simulink model "testing_stuff_ej2"  (R2023b)
settings: Solver=VariableStepAuto  StartTime=0.0  StopTime=0.1  FixedStep=step  RelTol=1e-3
values from neighbouring files (symbols this model uses):
  ej3_offset = 1e-5    (= 1e-05)    [EJ3.m]
  fd = 10    [EJ3.m]
  Kenv = 1000000    [EJ3.m]
  Kp = wn^2    (= 21268.5764063)    [EJ3.m]
  Kpf = 160000*1000    (= 160000000)    [EJ3.m]
  Kv = eta*(2*sqrt(Kp))    [EJ3.m]
  Kvf = 800*sqrt(1000)    [EJ3.m]
  mask = [1 1 0 0 0 0]    [EJ3.m]
  q0 = [pi/2,-pi/2]    [EJ3.m]
  robot = SerialLink(L, 'tool', Tool)    [EJ3.m]
  WO_R2x2 = WO_T(1:2,1:2)    [EJ3.m]
  WO_T = trotz(-pi/4)*transl(-1,-1,0)    [EJ3.m]
undefined symbols (not defined in the file or in its folder): coriolis, fkine, friction, gravload, inertia, jacob0, subsref, transl
libraries: roblocks x2, matrix_library x2
settings Model: Creator=alero  LastModifiedBy=alero

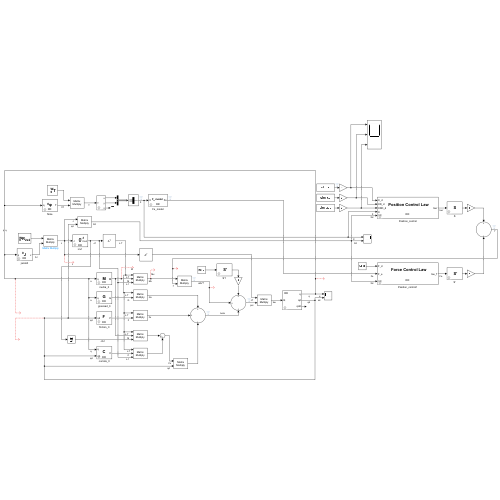
[thumbnail: Simulink's stored preview of the top-level diagram]
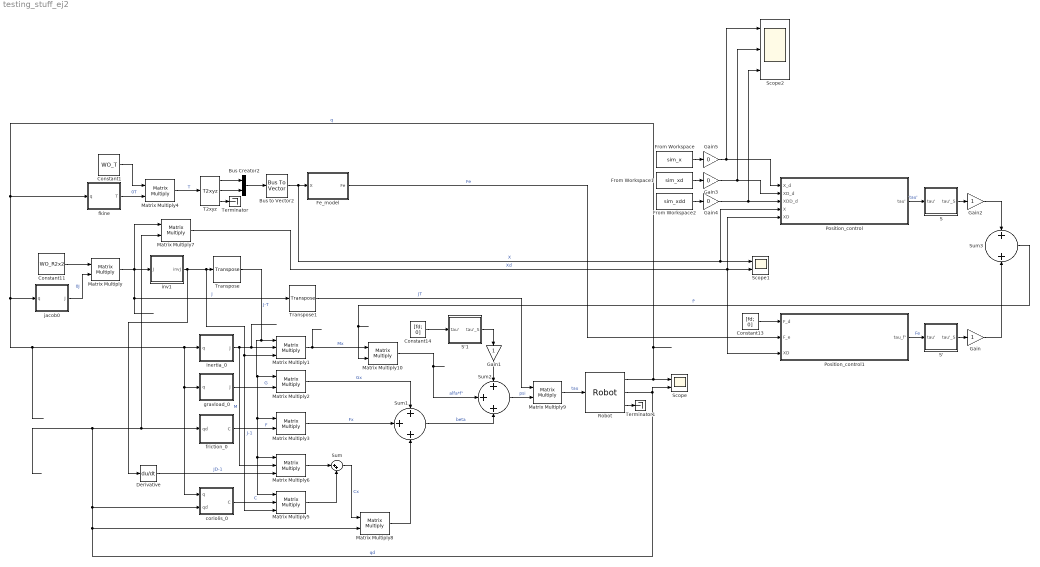
== system testing_stuff_ej2 ==
  Bus Creator2 : BusCreator  Inputs=2
  Bus to Vector2 : BusToVector
  Constant1 : Constant  Value=WO_T  VectorParams1D=off
      mask Display:
      | text(0.35, 0.8, '\bf\fontsize{16}^W_0T', 'texmode', 'on', 'verticalAlignment', 'top', 'horizontalAlignment', 'left')
      | %text(0.45, 0.65, '\fontsize{10}0', 'texmode', 'on','verticalAlignment', 'bottom', 'horizontalAlignment', 'right')
  Constant11 : Constant  Value=WO_R2x2  VectorParams1D=off
      mask Display:
      | text(0.1, 0.8, '\bf\fontsize{16}^W_0R_{2x2}', 'texmode', 'on', 'verticalAlignment', 'top', 'horizontalAlignment', 'left')
      | %text(0.45, 0.65, '\fontsize{10}0', 'texmode', 'on','verticalAlignment', 'bottom', 'horizontalAlignment', 'right')
  Constant13 : Constant  Value=[fd; 0]
  Constant14 : Constant  Value=[fd; 0]
  Derivative : Derivative
  Fe_model : Subsystem  mask{robot=robot}
      mask prompts: robot "Robot object"
      mask help: Robot forward kinematics.
      mask Help:
      | Compute homogeneous transform for robot end-effector given joint coordinates
      | 
      | 
      | <b>Parameters::</b>
      | 
      | Robot (SerialLink class)  The N-axis robot object for computing forward kinematics.
      | 
      | <b>Inputs::</b>
      | 
      | q (1xN) joint coordinates
      | 
      | <b>Outputs::</b>
      | 
      | T (4x4) the pose of the end effector as a homogeneous transformation
      | 
      | <b>Notes::</b>
      | 
      | - A wrapper for the Toolbox method fkine().
      mask Display:
      | text(0.2, 0.8, '\bf\fontsize{10}F_e model', 'texmode', 'on', 'verticalAlignment', 'top', 'horizontalAlignment', 'left')
      | %text(0.45, 0.65, '\fontsize{10}0', 'texmode', 'on','verticalAlignment', 'bottom', 'horizontalAlignment', 'right')
      | if ~isempty(robot)
      |     text(0.5, 0.2, robot.name,  'horizontalAlignment', 'center')
      | end
      | port_label('input', 1, 'X')
      | port_label('output', 1, 'Fe')
  From Workspace : FromWorkspace  VariableName=sim_x  SampleTime=step
  From Workspace1 : FromWorkspace  VariableName=sim_xd  SampleTime=step
  From Workspace2 : FromWorkspace  VariableName=sim_xdd  SampleTime=step
  Gain : Gain
  Gain1 : Gain
  Gain2 : Gain
  Gain3 : Gain  Gain=0
  Gain4 : Gain  Gain=0
  Gain5 : Gain  Gain=0
  Matrix Multiply{,2..4,7..10} (8 alike) : Product  Multiplication=Matrix(*)
  Matrix Multiply1 : Product  Inputs=3  Multiplication=Matrix(*)
  Matrix Multiply5 : Product  Inputs=3  Multiplication=Matrix(*)
  Matrix Multiply6 : Product  Inputs=3  Multiplication=Matrix(*)
  Position_control : Subsystem  mask{robot=robot}
      mask prompts: robot "Robot object"
      mask help: Robot forward kinematics.
      mask Help:
      | Compute homogeneous transform for robot end-effector given joint coordinates
      | 
      | 
      | <b>Parameters::</b>
      | 
      | Robot (SerialLink class)  The N-axis robot object for computing forward kinematics.
      | 
      | <b>Inputs::</b>
      | 
      | q (1xN) joint coordinates
      | 
      | <b>Outputs::</b>
      | 
      | T (4x4) the pose of the end effector as a homogeneous transformation
      | 
      | <b>Notes::</b>
      | 
      | - A wrapper for the Toolbox method fkine().
      mask Display:
      | text(0.18, 0.8, '\bf\fontsize{16}Position Control Law', 'texmode', 'on', 'verticalAlignment', 'top', 'horizontalAlignment', 'left')
      | %text(0.45, 0.65, '\fontsize{10}0', 'texmode', 'on','verticalAlignment', 'bottom', 'horizontalAlignment', 'right')
      | if ~isempty(robot)
      |     text(0.5, 0.2, robot.name,  'horizontalAlignment', 'center')
      | end
      | port_label('input', 1, 'X_d')
      | port_label('input', 2, 'XD_d')
      | port_label('input', 3, 'XDD_d')
      | port_label('input', 4, 'X')
      | port_label('input', 5, 'XD')
      | port_label('output', 1, 'tau''')
  Position_control1 : Subsystem  mask{robot=robot}
      mask prompts: robot "Robot object"
      mask help: Robot forward kinematics.
      mask Help:
      | Compute homogeneous transform for robot end-effector given joint coordinates
      | 
      | 
      | <b>Parameters::</b>
      | 
      | Robot (SerialLink class)  The N-axis robot object for computing forward kinematics.
      | 
      | <b>Inputs::</b>
      | 
      | q (1xN) joint coordinates
      | 
      | <b>Outputs::</b>
      | 
      | T (4x4) the pose of the end effector as a homogeneous transformation
      | 
      | <b>Notes::</b>
      | 
      | - A wrapper for the Toolbox method fkine().
      mask Display:
      | text(0.23, 0.8, '\bf\fontsize{16}Force Control Law', 'texmode', 'on', 'verticalAlignment', 'top', 'horizontalAlignment', 'left')
      | %text(0.45, 0.65, '\fontsize{10}0', 'texmode', 'on','verticalAlignment', 'bottom', 'horizontalAlignment', 'right')
      | if ~isempty(robot)
      |     text(0.5, 0.2, robot.name,  'horizontalAlignment', 'center')
      | end
      | port_label('input', 1, 'F_d')
      | port_label('input', 2, 'F_e')
      | port_label('input', 3, 'XD')
      | port_label('output', 1, 'tau_f''')
  Robot : roblocks/Arm/Robot  robot=robot  q0=robot.ikine(transl(1+sqrt(1/2)*ej3_offset,1+sqrt(1/2)*ej3_offset,0), 'q0',q0,'mask',mask)
  S : Subsystem  mask{robot=robot}
      mask prompts: robot "Robot object"
      mask help: Robot Jacobian in world coordinates
      mask init:
      | if ~isempty(robot)
      |     n=robot.n;
      | end
      mask Help:
      | Jacobian matrix relating joint coordinate rates to end-effector spatial
      | velocity expressed in the world frame.
      | 
      | <b>Parameters::</b>
      | 
      | Robot (SerialLink class)  The N-axis robot object for which the Jacobian is
      |                           computed.
      | 
      | <b>Inputs::</b>
      | 
      | q (1xN) joint coordinates
      | 
      | <b>Outputs::</b>
      | 
      | J (6xN) the Jacobian matrix
      | 
      | <b>Notes::</b>
      | 
      | - A wrapper for the Toolbox method jacob0().
      mask Display:
      | text(0.45, 0.75, '\bf\fontsize{16}S', 'texmode', 'on', 'verticalAlignment', 'top', 'horizontalAlignment', 'left')
      | %text(0.45, 0.65, '\fontsize{10}0', 'texmode', 'on','verticalAlignment', 'bottom', 'horizontalAlignment', 'right')
      | if ~isempty(robot)
      |     %text(0.5, 0.2, robot.name,  'horizontalAlignment', 'center')
      | end
      | %port_label('input', 1, 'J')
      | %port_label('output', 1, 'invJ')
  S' : Subsystem  mask{robot=robot}
      mask prompts: robot "Robot object"
      mask help: Robot Jacobian in world coordinates
      mask init:
      | if ~isempty(robot)
      |     n=robot.n;
      | end
      mask Help:
      | Jacobian matrix relating joint coordinate rates to end-effector spatial
      | velocity expressed in the world frame.
      | 
      | <b>Parameters::</b>
      | 
      | Robot (SerialLink class)  The N-axis robot object for which the Jacobian is
      |                           computed.
      | 
      | <b>Inputs::</b>
      | 
      | q (1xN) joint coordinates
      | 
      | <b>Outputs::</b>
      | 
      | J (6xN) the Jacobian matrix
      | 
      | <b>Notes::</b>
      | 
      | - A wrapper for the Toolbox method jacob0().
      mask Display:
      | text(0.45, 0.75, '\bf\fontsize{16}S''', 'texmode', 'on', 'verticalAlignment', 'top', 'horizontalAlignment', 'left')
      | %text(0.45, 0.65, '\fontsize{10}0', 'texmode', 'on','verticalAlignment', 'bottom', 'horizontalAlignment', 'right')
      | if ~isempty(robot)
      |     %text(0.5, 0.2, robot.name,  'horizontalAlignment', 'center')
      | end
      | %port_label('input', 1, 'J')
      | %port_label('output', 1, 'invJ')
  S'1 : Subsystem  mask{robot=robot}
      mask prompts: robot "Robot object"
      mask help: Robot Jacobian in world coordinates
      mask init:
      | if ~isempty(robot)
      |     n=robot.n;
      | end
      mask Help:
      | Jacobian matrix relating joint coordinate rates to end-effector spatial
      | velocity expressed in the world frame.
      | 
      | <b>Parameters::</b>
      | 
      | Robot (SerialLink class)  The N-axis robot object for which the Jacobian is
      |                           computed.
      | 
      | <b>Inputs::</b>
      | 
      | q (1xN) joint coordinates
      | 
      | <b>Outputs::</b>
      | 
      | J (6xN) the Jacobian matrix
      | 
      | <b>Notes::</b>
      | 
      | - A wrapper for the Toolbox method jacob0().
      mask Display:
      | text(0.45, 0.75, '\bf\fontsize{16}S''', 'texmode', 'on', 'verticalAlignment', 'top', 'horizontalAlignment', 'left')
      | %text(0.45, 0.65, '\fontsize{10}0', 'texmode', 'on','verticalAlignment', 'bottom', 'horizontalAlignment', 'right')
      | if ~isempty(robot)
      |     %text(0.5, 0.2, robot.name,  'horizontalAlignment', 'center')
      | end
      | %port_label('input', 1, 'J')
      | %port_label('output', 1, 'invJ')
  Scope : Scope  NumInputPorts=2
  Scope1 : Scope  NumInputPorts=2
  Scope2 : Scope  NumInputPorts=3
  Sum : Sum  Inputs=|++
  Sum1 : Sum  Inputs=+++
  Sum2 : Sum  Inputs=+++
  Sum3 : Sum  Inputs=+|+
  T2xyz : roblocks/Toolbox/T2xyz
  Terminator : Terminator
  Terminator1 : Terminator
  Transpose : matrix_library/Transpose
  Transpose1 : matrix_library/Transpose
  coriolis_0 : Subsystem  mask{robot=robot}
      mask prompts: robot "Robot object"
      mask help: Robot Jacobian in world coordinates
      mask init:
      | if ~isempty(robot)
      |     n=robot.n;
      | end
      mask Help:
      | Jacobian matrix relating joint coordinate rates to end-effector spatial
      | velocity expressed in the world frame.
      | 
      | <b>Parameters::</b>
      | 
      | Robot (SerialLink class)  The N-axis robot object for which the Jacobian is
      |                           computed.
      | 
      | <b>Inputs::</b>
      | 
      | q (1xN) joint coordinates
      | 
      | <b>Outputs::</b>
      | 
      | J (6xN) the Jacobian matrix
      | 
      | <b>Notes::</b>
      | 
      | - A wrapper for the Toolbox method jacob0().
      mask Display:
      | text(0.4, 0.8, '\bf\fontsize{16}C', 'texmode', 'on', 'verticalAlignment', 'top', 'horizontalAlignment', 'left')
      | %text(0.45, 0.65, '\fontsize{10}0', 'texmode', 'on','verticalAlignment', 'bottom', 'horizontalAlignment', 'right')
      | if ~isempty(robot)
      |     text(0.5, 0.2, robot.name,  'horizontalAlignment', 'center')
      | end
      | port_label('input', 1, 'q')
      | port_label('output', 1, 'C')
      | port_label('input',2,'qd')
  fkine : Subsystem  mask{robot=robot}
      mask prompts: robot "Robot object"
      mask help: Robot forward kinematics.
      mask Help:
      | Compute homogeneous transform for robot end-effector given joint coordinates
      | 
      | 
      | <b>Parameters::</b>
      | 
      | Robot (SerialLink class)  The N-axis robot object for computing forward kinematics.
      | 
      | <b>Inputs::</b>
      | 
      | q (1xN) joint coordinates
      | 
      | <b>Outputs::</b>
      | 
      | T (4x4) the pose of the end effector as a homogeneous transformation
      | 
      | <b>Notes::</b>
      | 
      | - A wrapper for the Toolbox method fkine().
      mask Display:
      | text(0.35, 0.8, '\bf\fontsize{16}^0\phi', 'texmode', 'on', 'verticalAlignment', 'top', 'horizontalAlignment', 'left')
      | %text(0.45, 0.65, '\fontsize{10}0', 'texmode', 'on','verticalAlignment', 'bottom', 'horizontalAlignment', 'right')
      | if ~isempty(robot)
      |     text(0.5, 0.2, robot.name,  'horizontalAlignment', 'center')
      | end
      | port_label('input', 1, 'q')
      | port_label('output', 1, 'T')
  friction_0 : Subsystem  mask{robot=robot}
      mask prompts: robot "Robot object"
      mask help: Robot Jacobian in world coordinates
      mask init:
      | if ~isempty(robot)
      |     n=robot.n;
      | end
      mask Help:
      | Jacobian matrix relating joint coordinate rates to end-effector spatial
      | velocity expressed in the world frame.
      | 
      | <b>Parameters::</b>
      | 
      | Robot (SerialLink class)  The N-axis robot object for which the Jacobian is
      |                           computed.
      | 
      | <b>Inputs::</b>
      | 
      | q (1xN) joint coordinates
      | 
      | <b>Outputs::</b>
      | 
      | J (6xN) the Jacobian matrix
      | 
      | <b>Notes::</b>
      | 
      | - A wrapper for the Toolbox method jacob0().
      mask Display:
      | text(0.4, 0.8, '\bf\fontsize{16}F', 'texmode', 'on', 'verticalAlignment', 'top', 'horizontalAlignment', 'left')
      | %text(0.45, 0.65, '\fontsize{10}0', 'texmode', 'on','verticalAlignment', 'bottom', 'horizontalAlignment', 'right')
      | if ~isempty(robot)
      |     text(0.5, 0.2, robot.name,  'horizontalAlignment', 'center')
      | end
      | port_label('input', 1, 'qd')
      | port_label('output', 1, 'F')
  gravload_0 : Subsystem  mask{robot=robot}
      mask prompts: robot "Robot object"
      mask help: Robot Jacobian in world coordinates
      mask init:
      | if ~isempty(robot)
      |     n=robot.n;
      | end
      mask Help:
      | Jacobian matrix relating joint coordinate rates to end-effector spatial
      | velocity expressed in the world frame.
      | 
      | <b>Parameters::</b>
      | 
      | Robot (SerialLink class)  The N-axis robot object for which the Jacobian is
      |                           computed.
      | 
      | <b>Inputs::</b>
      | 
      | q (1xN) joint coordinates
      | 
      | <b>Outputs::</b>
      | 
      | J (6xN) the Jacobian matrix
      | 
      | <b>Notes::</b>
      | 
      | - A wrapper for the Toolbox method jacob0().
      mask Display:
      | text(0.4, 0.8, '\bf\fontsize{16}G', 'texmode', 'on', 'verticalAlignment', 'top', 'horizontalAlignment', 'left')
      | %text(0.45, 0.65, '\fontsize{10}0', 'texmode', 'on','verticalAlignment', 'bottom', 'horizontalAlignment', 'right')
      | if ~isempty(robot)
      |     text(0.5, 0.2, robot.name,  'horizontalAlignment', 'center')
      | end
      | port_label('input', 1, 'q')
      | port_label('output', 1, 'G')
  inertia_0 : Subsystem  mask{robot=robot}
      mask prompts: robot "Robot object"
      mask help: Robot Jacobian in world coordinates
      mask init:
      | if ~isempty(robot)
      |     n=robot.n;
      | end
      mask Help:
      | Jacobian matrix relating joint coordinate rates to end-effector spatial
      | velocity expressed in the world frame.
      | 
      | <b>Parameters::</b>
      | 
      | Robot (SerialLink class)  The N-axis robot object for which the Jacobian is
      |                           computed.
      | 
      | <b>Inputs::</b>
      | 
      | q (1xN) joint coordinates
      | 
      | <b>Outputs::</b>
      | 
      | J (6xN) the Jacobian matrix
      | 
      | <b>Notes::</b>
      | 
      | - A wrapper for the Toolbox method jacob0().
      mask Display:
      | text(0.4, 0.8, '\bf\fontsize{16}M', 'texmode', 'on', 'verticalAlignment', 'top', 'horizontalAlignment', 'left')
      | %text(0.45, 0.65, '\fontsize{10}0', 'texmode', 'on','verticalAlignment', 'bottom', 'horizontalAlignment', 'right')
      | if ~isempty(robot)
      |     text(0.5, 0.2, robot.name,  'horizontalAlignment', 'center')
      | end
      | port_label('input', 1, 'q')
      | port_label('output', 1, 'M')
  inv1 : Subsystem  mask{robot=robot}
      mask prompts: robot "Robot object"
      mask help: Robot Jacobian in world coordinates
      mask init:
      | if ~isempty(robot)
      |     n=robot.n;
      | end
      mask Help:
      | Jacobian matrix relating joint coordinate rates to end-effector spatial
      | velocity expressed in the world frame.
      | 
      | <b>Parameters::</b>
      | 
      | Robot (SerialLink class)  The N-axis robot object for which the Jacobian is
      |                           computed.
      | 
      | <b>Inputs::</b>
      | 
      | q (1xN) joint coordinates
      | 
      | <b>Outputs::</b>
      | 
      | J (6xN) the Jacobian matrix
      | 
      | <b>Notes::</b>
      | 
      | - A wrapper for the Toolbox method jacob0().
      mask Display:
      | text(0.4, 0.9, '\bf\fontsize{16}\{\}^{-1}', 'texmode', 'on', 'verticalAlignment', 'top', 'horizontalAlignment', 'left')
      | %text(0.45, 0.65, '\fontsize{10}0', 'texmode', 'on','verticalAlignment', 'bottom', 'horizontalAlignment', 'right')
      | if ~isempty(robot)
      |     text(0.5, 0.2, robot.name,  'horizontalAlignment', 'center')
      | end
      | port_label('input', 1, 'J')
      | port_label('output', 1, 'invJ')
  "jacob0 " : Subsystem  mask{robot=robot}
      mask prompts: robot "Robot object"
      mask help: Robot Jacobian in world coordinates
      mask init:
      | if ~isempty(robot)
      |     n=robot.n;
      | end
      mask Help:
      | Jacobian matrix relating joint coordinate rates to end-effector spatial
      | velocity expressed in the world frame.
      | 
      | <b>Parameters::</b>
      | 
      | Robot (SerialLink class)  The N-axis robot object for which the Jacobian is
      |                           computed.
      | 
      | <b>Inputs::</b>
      | 
      | q (1xN) joint coordinates
      | 
      | <b>Outputs::</b>
      | 
      | J (6xN) the Jacobian matrix
      | 
      | <b>Notes::</b>
      | 
      | - A wrapper for the Toolbox method jacob0().
      mask Display:
      | text(0.35, 0.8, '\bf\fontsize{16}^0J', 'texmode', 'on', 'verticalAlignment', 'top', 'horizontalAlignment', 'left')
      | %text(0.45, 0.65, '\fontsize{10}0', 'texmode', 'on','verticalAlignment', 'bottom', 'horizontalAlignment', 'right')
      | if ~isempty(robot)
      |     text(0.5, 0.2, robot.name,  'horizontalAlignment', 'center')
      | end
      | port_label('input', 1, 'q')
      | port_label('output', 1, 'J')
  wires:
  "jacob0 "/1(J) -> Matrix Multiply/2  "0J"
  Constant11/1 -> Matrix Multiply/1
  Matrix Multiply/1 -> Transpose1/1, Matrix Multiply7/1, inv1/1(J)  "J"
  inv1/1(invJ) -> Derivative/1, Matrix Multiply1/3, Matrix Multiply5/3, Transpose/1  "J-1"
  Transpose/1 -> Matrix Multiply6/1, Matrix Multiply5/1, Matrix Multiply3/1, Matrix Multiply2/1, Matrix Multiply1/1  "J-T"
  inertia_0/1(J) -> Matrix Multiply6/2, Matrix Multiply1/2  "M"
  Matrix Multiply1/1 -> Matrix Multiply10/1  "Mx"
  gravload_0/1(J) -> Matrix Multiply2/2  "G"
  Matrix Multiply2/1 -> Sum1/1  "Gx"
  Matrix Multiply3/1 -> Sum1/2  "Fx"
  friction_0/1(C) -> Matrix Multiply3/2  "F"
  T2xyz/2 -> Bus Creator2/2
  Bus Creator2/1 -> Bus to Vector2/1
  T2xyz/1 -> Bus Creator2/1
  Matrix Multiply4/1 -> T2xyz/1  "T"
  Constant1/1 -> Matrix Multiply4/1
  fkine/1(T) -> Matrix Multiply4/2  "0T"
  T2xyz/3 -> Terminator/1
  Bus to Vector2/1 -> Position_control/4(X), Scope1/1, Fe_model/1(X)  "X"
  Fe_model/1(Fe) -> Position_control1/2(F_e)  "Fe"
  Matrix Multiply5/1 -> Sum/2
  coriolis_0/1(C) -> Matrix Multiply5/2  "C"
  Matrix Multiply6/1 -> Sum/1
  Sum/1 -> Matrix Multiply8/1  "Cx"
  Matrix Multiply7/1 -> Position_control1/3(XD), Position_control/5(XD), Scope1/2  "Xd"
  Matrix Multiply8/1 -> Sum1/3
  Sum1/1 -> Sum2/3  "beta"
  S'1/1(tau'_S) -> Gain1/1
  Matrix Multiply10/1 -> Sum2/2  "alfa*f'"
  Matrix Multiply9/1 -> Robot/1  "tau"
  Sum2/1 -> Matrix Multiply9/2  "psi"
  Transpose1/1 -> Matrix Multiply9/1  "JT"
  Robot/1 -> Scope/1, "jacob0 "/1(q), coriolis_0/1(q), gravload_0/1(q), inertia_0/1(q), fkine/1(q)  "q"
  Robot/2 -> Scope/2, Matrix Multiply7/2, friction_0/1(qd), coriolis_0/2(qd), Matrix Multiply8/2  "qd"
  Robot/3 -> Terminator1/1
  From Workspace/1 -> Gain5/1
  From Workspace1/1 -> Gain3/1
  From Workspace2/1 -> Gain4/1
  Constant13/1 -> Position_control1/1(F_d)
  Position_control/1(tau') -> S/1(tau')  "tau'"
  S/1(tau'_S) -> Gain2/1
  Position_control1/1(tau_f') -> S'/1(tau')  "Fe"
  S'/1(tau'_S) -> Gain/1
  Sum3/1 -> Matrix Multiply10/2  "f'"
  Constant14/1 -> S'1/1(tau')
  Derivative/1 -> Matrix Multiply6/3  "JD-1"
  Gain/1 -> Sum3/2
  Gain1/1 -> Sum2/1
  Gain2/1 -> Sum3/1
  Gain3/1 -> Position_control/2(XD_d), Scope2/2
  Gain4/1 -> Position_control/3(XDD_d), Scope2/3
  Gain5/1 -> Position_control/1(X_d), Scope2/1

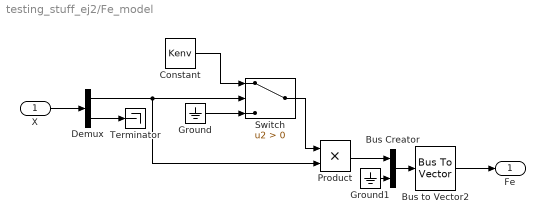
== system testing_stuff_ej2/Fe_model ==
  X : Inport
  Bus Creator : BusCreator  Inputs=2
  Bus to Vector2 : BusToVector
  Constant : Constant  Value=Kenv
  Demux : Demux  Outputs=2
  Ground : Ground
  Ground1 : Ground
  Product : Product
  Switch : Switch  Criteria=u2 > Threshold  SaturateOnIntegerOverflow=off  InputSameDT=off
  Terminator : Terminator
  Fe : Outport  VectorParamsAs1DForOutWhenUnconnected=off
  wires:
  X/1 -> Demux/1
  Demux/2 -> Terminator/1
  Demux/1 -> Switch/2, Product/2
  Switch/1 -> Product/1
  Constant/1 -> Switch/1
  Ground/1 -> Switch/3
  Ground1/1 -> Bus Creator/2
  Bus Creator/1 -> Bus to Vector2/1
  Product/1 -> Bus Creator/1
  Bus to Vector2/1 -> Fe/1

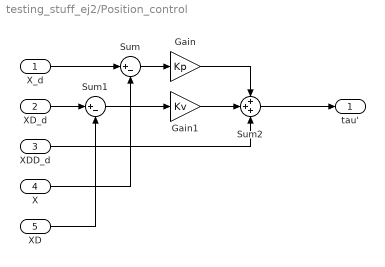
== system testing_stuff_ej2/Position_control ==
  X_d : Inport
  XD_d : Inport  Port=2
  XDD_d : Inport  Port=3
  X : Inport  Port=4
  XD : Inport  Port=5
  Gain : Gain  Gain=Kp
  Gain1 : Gain  Gain=Kv
  Sum : Sum  Inputs=|+-
  Sum1 : Sum  Inputs=|+-
  Sum2 : Sum  Inputs=+++
  tau' : Outport  VectorParamsAs1DForOutWhenUnconnected=off
  wires:
  X_d/1 -> Sum/1
  XD_d/1 -> Sum1/1
  X/1 -> Sum/2
  XD/1 -> Sum1/2
  Sum1/1 -> Gain1/1
  Sum/1 -> Gain/1
  Gain/1 -> Sum2/1
  Gain1/1 -> Sum2/2
  XDD_d/1 -> Sum2/3
  Sum2/1 -> tau'/1

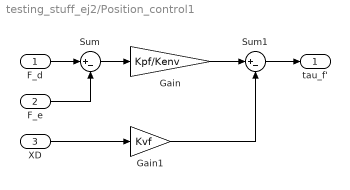
== system testing_stuff_ej2/Position_control1 ==
  F_d : Inport
  F_e : Inport  Port=2
  XD : Inport  Port=3
  Gain : Gain  Gain=Kpf/Kenv
  Gain1 : Gain  Gain=Kvf
  Sum : Sum  Inputs=|+-
  Sum1 : Sum  Inputs=|+-
  tau_f' : Outport  VectorParamsAs1DForOutWhenUnconnected=off
  wires:
  F_d/1 -> Sum/1
  F_e/1 -> Sum/2
  Sum/1 -> Gain/1
  XD/1 -> Gain1/1
  Gain/1 -> Sum1/1
  Gain1/1 -> Sum1/2
  Sum1/1 -> tau_f'/1

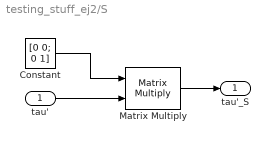
== system testing_stuff_ej2/S ==
  tau' : Inport
  Constant : Constant  Value=[0 0; 0 1]
  Matrix Multiply : Product  Multiplication=Matrix(*)
  tau'_S : Outport  VectorParamsAs1DForOutWhenUnconnected=off
  wires:
  tau'/1 -> Matrix Multiply/2
  Matrix Multiply/1 -> tau'_S/1
  Constant/1 -> Matrix Multiply/1

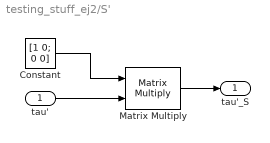
== system testing_stuff_ej2/S' ==
  tau' : Inport
  Constant : Constant  Value=[1 0; 0 0]
  Matrix Multiply : Product  Multiplication=Matrix(*)
  tau'_S : Outport  VectorParamsAs1DForOutWhenUnconnected=off
  wires:
  tau'/1 -> Matrix Multiply/2
  Matrix Multiply/1 -> tau'_S/1
  Constant/1 -> Matrix Multiply/1

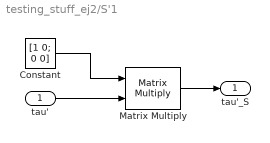
== system testing_stuff_ej2/S'1 ==
  tau' : Inport
  Constant : Constant  Value=[1 0; 0 0]
  Matrix Multiply : Product  Multiplication=Matrix(*)
  tau'_S : Outport  VectorParamsAs1DForOutWhenUnconnected=off
  wires:
  tau'/1 -> Matrix Multiply/2
  Matrix Multiply/1 -> tau'_S/1
  Constant/1 -> Matrix Multiply/1

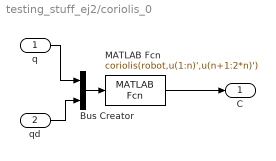
== system testing_stuff_ej2/coriolis_0 ==
  q : Inport
  qd : Inport  Port=2
  Bus Creator : BusCreator  Inputs=2
  MATLAB Fcn : MATLABFcn  MATLABFcn=coriolis(robot,u(1:n)',u(n+1:2*n)')  OutputDimensions=[robot.n robot.n]  Output1D=off
  C : Outport  VectorParamsAs1DForOutWhenUnconnected=off
  wires:
  MATLAB Fcn/1 -> C/1
  Bus Creator/1 -> MATLAB Fcn/1
  q/1 -> Bus Creator/1
  qd/1 -> Bus Creator/2

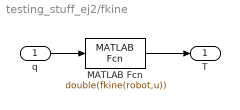
== system testing_stuff_ej2/fkine ==
  q : Inport
  MATLAB Fcn : MATLABFcn  MATLABFcn=double(fkine(robot,u))  OutputDimensions=[4 4]  Output1D=off
  T : Outport  VectorParamsAs1DForOutWhenUnconnected=off
  wires:
  q/1 -> MATLAB Fcn/1
  MATLAB Fcn/1 -> T/1

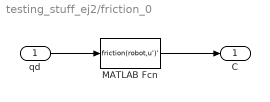
== system testing_stuff_ej2/friction_0 ==
  qd : Inport
  MATLAB Fcn : MATLABFcn  MATLABFcn=friction(robot,u')'  OutputDimensions=[robot.n 1]  Output1D=off
  C : Outport  VectorParamsAs1DForOutWhenUnconnected=off
  wires:
  MATLAB Fcn/1 -> C/1
  qd/1 -> MATLAB Fcn/1

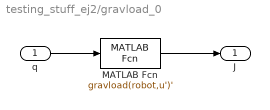
== system testing_stuff_ej2/gravload_0 ==
  q : Inport
  MATLAB Fcn : MATLABFcn  MATLABFcn=gravload(robot,u')'  OutputDimensions=[robot.n 1]  Output1D=off
  J : Outport  VectorParamsAs1DForOutWhenUnconnected=off
  wires:
  MATLAB Fcn/1 -> J/1
  q/1 -> MATLAB Fcn/1

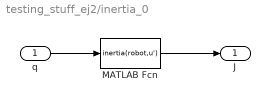
== system testing_stuff_ej2/inertia_0 ==
  q : Inport
  MATLAB Fcn : MATLABFcn  MATLABFcn=inertia(robot,u')  OutputDimensions=[robot.n robot.n]  Output1D=off
  J : Outport  VectorParamsAs1DForOutWhenUnconnected=off
  wires:
  MATLAB Fcn/1 -> J/1
  q/1 -> MATLAB Fcn/1

== system testing_stuff_ej2/inv1 ==
  J : Inport
  MATLAB Fcn : MATLABFcn  MATLABFcn=inv(u)  OutputDimensions=[n n]  Output1D=off
  invJ : Outport  VectorParamsAs1DForOutWhenUnconnected=off
  wires:
  MATLAB Fcn/1 -> invJ/1
  J/1 -> MATLAB Fcn/1

== system testing_stuff_ej2/jacob0  ==
  q : Inport
  MATLAB Fcn : MATLABFcn  MATLABFcn=subsref(jacob0(robot,u), struct('type', '()', 'subs', {{1:2, 1:2}}));  OutputDimensions=[n n]  Output1D=off
  J : Outport  VectorParamsAs1DForOutWhenUnconnected=off
  wires:
  MATLAB Fcn/1 -> J/1
  q/1 -> MATLAB Fcn/1
